simulink model "HighLevelController"  (R2023a)
settings: Solver=VariableStepAuto  StartTime=0.0  StopTime=10.0  RelTol=1e-3
settings Model: Creator=Сафроновы  LastModifiedBy=Сафроновы

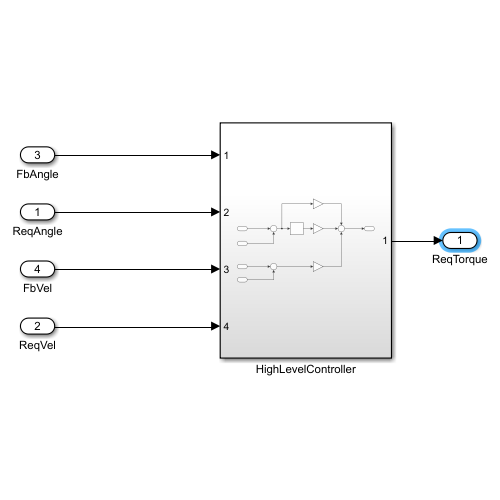
[thumbnail: Simulink's stored preview of the top-level diagram]
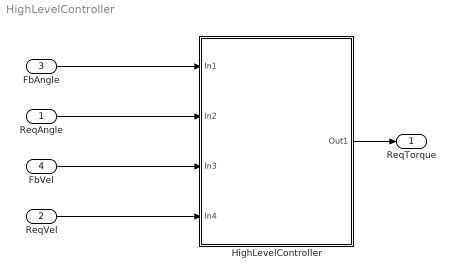
== system HighLevelController ==
  ReqAngle : Inport
  ReqVel : Inport  Port=2
  FbAngle : Inport  Port=3
  FbVel : Inport  Port=4
  HighLevelController : Subsystem
  ReqTorque : Outport
  wires:
  FbAngle/1 -> HighLevelController/1(In1)
  ReqAngle/1 -> HighLevelController/2(In2)
  FbVel/1 -> HighLevelController/3(In3)
  ReqVel/1 -> HighLevelController/4(In4)
  HighLevelController/1(Out1) -> ReqTorque/1

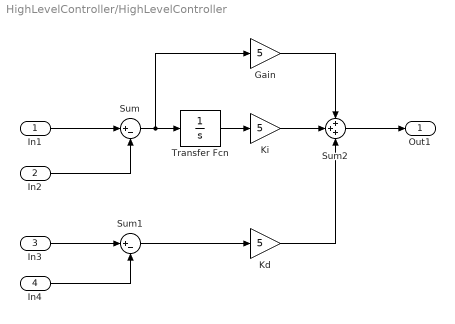
== system HighLevelController/HighLevelController ==
  In1 : Inport
  In2 : Inport  Port=2
  In3 : Inport  Port=3
  In4 : Inport  Port=4
  Gain : Gain  Gain=5
  Kd : Gain  Gain=5
  Ki : Gain  Gain=5
  Sum : Sum  Inputs=|+-
  Sum1 : Sum  Inputs=|+-
  Sum2 : Sum  Inputs=+++
  Transfer Fcn : TransferFcn  Denominator=[1 0]
  Out1 : Outport
  wires:
  Ki/1 -> Sum2/2
  Sum/1 -> Gain/1, Transfer Fcn/1
  Kd/1 -> Sum2/3
  Gain/1 -> Sum2/1
  In4/1 -> Sum1/2
  In2/1 -> Sum/2
  Sum1/1 -> Kd/1
  Transfer Fcn/1 -> Ki/1
  Sum2/1 -> Out1/1
  In3/1 -> Sum1/1
  In1/1 -> Sum/1
